simulink model "Problem4"  (R2020b)
settings: Solver=VariableStepAuto  StartTime=0.0  StopTime=0.5  RelTol=1e-3
settings Model: Creator=hp  LastModifiedBy=hp

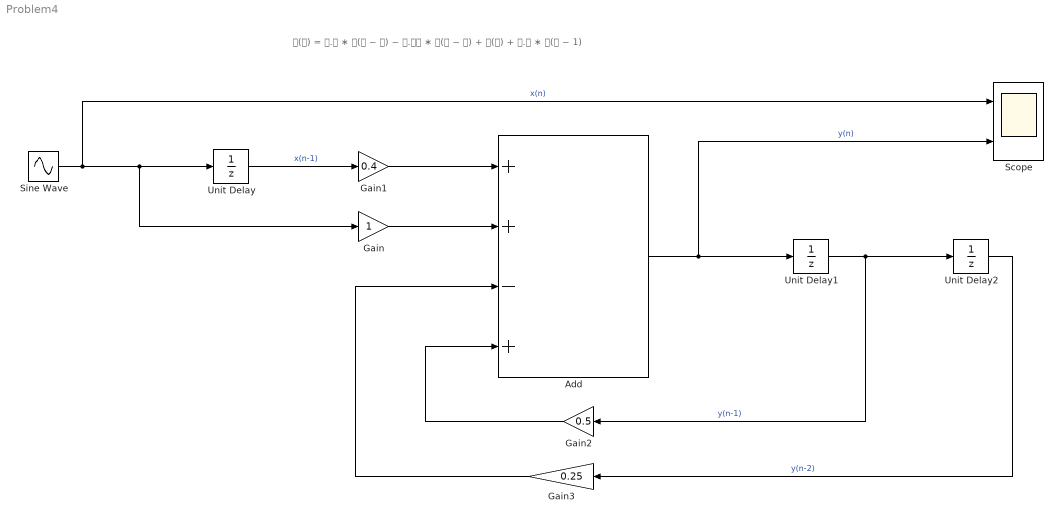
== system Problem4 ==
  note: 𝐲(𝐧) = 𝟎.𝟓 ∗ 𝐲(𝐧 − 𝟏) − 𝟎.𝟐𝟓 ∗ 𝐲(𝐧 − 𝟐) + 𝐱(𝐧) + 𝟎.𝟒 ∗ 𝐱(𝐧 − 1)
  Add : Sum  Inputs=++-+
  Gain : Gain
  Gain1 : Gain  Gain=0.4
  Gain2 : Gain  Gain=0.5
  Gain3 : Gain  Gain=0.25
  Scope : Scope  NumInputPorts=2
  Sine Wave : Sin  Frequency=50  SampleTime=0
  Unit Delay : UnitDelay  SampleTime=-1  HasFrameUpgradeWarning=on
  Unit Delay1 : UnitDelay  SampleTime=-1  HasFrameUpgradeWarning=on
  Unit Delay2 : UnitDelay  SampleTime=-1  HasFrameUpgradeWarning=on
  wires:
  Sine Wave/1 -> Scope/1, Gain/1, Unit Delay/1  "x(n)"
  Unit Delay/1 -> Gain1/1  "x(n-1)"
  Gain/1 -> Add/2
  Gain1/1 -> Add/1
  Add/1 -> Scope/2, Unit Delay1/1  "y(n)"
  Unit Delay1/1 -> Gain2/1, Unit Delay2/1  "y(n-1)"
  Gain2/1 -> Add/4
  Unit Delay2/1 -> Gain3/1  "y(n-2)"
  Gain3/1 -> Add/3
